simulink model "walkingRobot3DPath"  (R2022a)
settings: Solver=ode15s  StartTime=0.0  StopTime=70  RelTol=1e-2  EnableMultiTasking=on
PreLoadFcn:
  | robotParametersCtrl
values from neighbouring files (symbols this model uses):
  foot_x = 5    [robotParametersCtrl.m]
  foot_y = 4    [robotParametersCtrl.m]
  g = 9.80665    [robotParametersCtrl.m]
  h = 18    [robotParametersCtrl.m]
  Kwalk = 0.5    [robotParametersCtrl.m]
  stepHeight = 0.02    [robotParametersCtrl.m]
  torso_offset_z = -2    [robotParametersCtrl.m]
  TsCtrl = 0.05    [robotParametersCtrl.m]
  tWalk = 0.3    [robotParametersCtrl.m]
libraries: walkingRobotUtils x6, simulink x2, slpidlib x2
settings Model: Creator=scastro  LastModifiedBy=isamu
settings SolverCC: AlgebraicLoopSolver=TrustRegion
settings DataIOCC: ReturnWorkspaceOutputs=off  OutputTimes=0:0.01:10
settings OptimizationCC: LifeSpan=inf
settings DebuggingCC: UnconnectedInputMsg=warning  UnconnectedOutputMsg=warning  UnconnectedLineMsg=warning  AllowSymbolicDim=off  SFUnexpectedBacktrackingDiag=warning  SFNoUnconditionalDefaultTransitionDiag=warning  SFExecutionAtInitializationDiag=none  SFMachineParentedDataDiag=warning  UnitsInconsistencyMsg=none  ArithmeticOperatorsInVariantConditions=warning
settings SFSimCC: SimUseLocalCustomCode=off  CustomCodeUndefinedFunction=UseInterfaceOnly
settings RTWCC: RTWUseLocalCustomCode=off
settings CodeAppCC: StateflowObjectComments=on
settings GRTTargetCC: TargetLangStandard=C89/C90 (ANSI)
settings ConfigComp: CovMetricSettings=dw  CovSaveCumulativeToWorkspaceVar=on  CovSaveSingleToWorkspaceVar=on  CovExternalEMLEnable=off  CovSFcnEnable=off
settings SimscapeCC: SimscapeNormalizeSystem=off  SimscapeLogOpenViewer=on  SimscapeLogLimitData=off  SimscapeLogDataHistory=10000
settings ConfigurationSet: Description=SimMechanics 2G
settings DiagnosticsConfigSet: SimMechanicsRigidlyBoundBlock=none
settings ExplorerConfigSet: InternalSimMechanicsExplorerSettings="<ExplorerConfiguration><canonicalview>default</canonicalview><AnimationSetting><BasePlaybackSpeed>1.0</BasePlaybackSpeed><PlaybackSpeedFactor>1.0</PlaybackSpeedFactor></AnimationSetting><TilePanel><TileInfo><Tiles Columns=\"1\" Count=\"1\" Rows=\"1\"><Column Weight=\"1\"/><Row Weight=\"1\"/><Tile Height=\"1\" Width=\"1\" X=\"0\" Y=\"0\"/></Tiles></TileInfo><SceneInfo><SceneViewer><BGColor><R>0.60000002384185791</R><G>0.60000002384185791</G><B>0.60000002384185791</B></BGColor><Camera><DoPerspective>off</DoPerspective><Position><X>7.18002534815406079</X><Y>-8.21011991112170847</Y><Z>8.33180938462712462</Z></Position><Center><X>1.10741005252516134</X><Y>-0.176829942633513204</Y><Z>0.646464709811595872</Z></Center><Up><X>-0.335329266167064488</X><Y>0.506481739462631531</Y><Z>0.79437430147428989</Z></Up><ViewLimDist>1</ViewLimDist><YLim>0.739205014828661411</YLim><XLim>1.12849377732657596</XLim></Camera></SceneViewer></SceneInfo></TilePanel><MechEditorPanel><Cameras/><GfxPanelCameraMap/><VideoCreator><PlaybackSpeedRatio>1.0</PlaybackSpeedRatio><FrameRate>30</FrameRate><VideoFormat>Motion JPEG AVI</VideoFormat><FrameSize>auto</FrameSize></VideoCreator></MechEditorPanel></ExplorerConfiguration>"

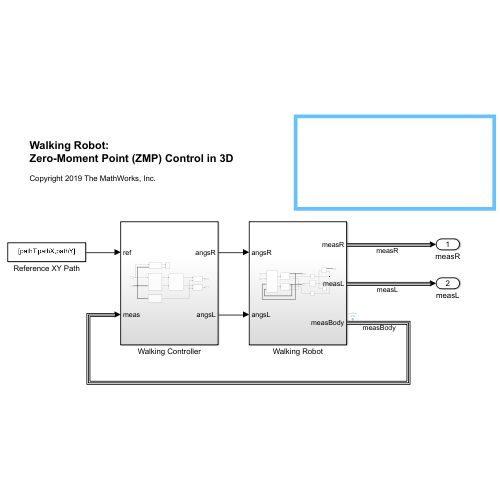
[thumbnail: Simulink's stored preview of the top-level diagram]
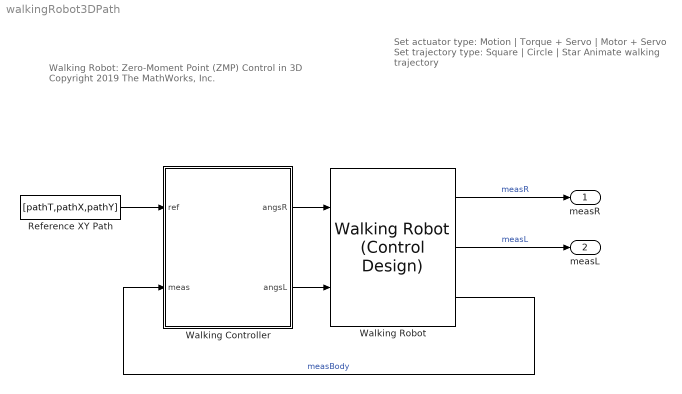
== system walkingRobot3DPath ==
  note: Set actuator type:
      | Motion | Torque + Servo | Motor + Servo
      |
      | Set trajectory type:
      | Square | Circle | Star
      |
      | Animate walking trajectory
  note: Walking Robot:
      | Zero-Moment Point (ZMP) Control in 3D
      |
      | Copyright 2019 The MathWorks, Inc.
  Reference XY Path : FromWorkspace  VariableName=[pathT,pathX,pathY]  SampleTime=TsCtrl  OutputAfterFinalValue=Holding final value
  Walking Controller : Subsystem
  Walking Robot : walkingRobotUtils/Walking Robot (Control Design)  SystemSampleTime=-1  VariantActivationTime=update diagram  Latency=0  AutoFrameSizeCalculation=off
  measR : Outport  VectorParamsAs1DForOutWhenUnconnected=off
  measL : Outport  Port=2  VectorParamsAs1DForOutWhenUnconnected=off
  wires:
  Walking Robot/1 -> measR/1  "measR"
  Walking Robot/2 -> measL/1  "measL"
  Walking Controller/1(angsR) -> Walking Robot/1
  Walking Controller/2(angsL) -> Walking Robot/2
  Walking Robot/3 -> Walking Controller/2(meas)  "measBody"
  Reference XY Path/1 -> Walking Controller/1(ref)

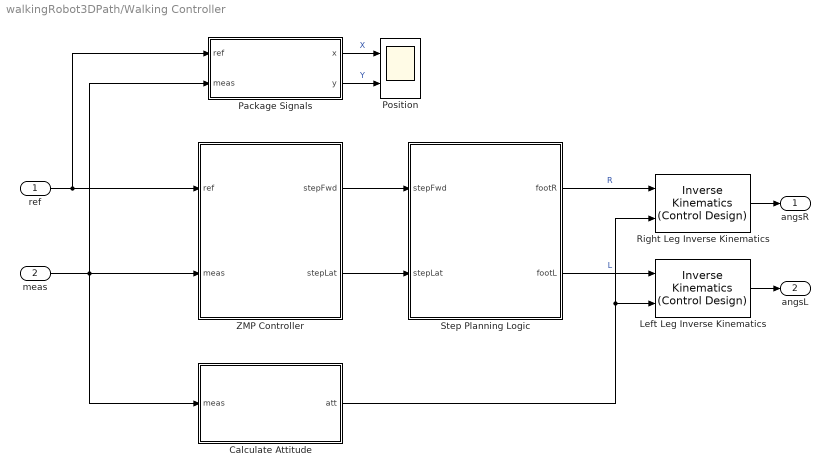
== system walkingRobot3DPath/Walking Controller ==
  ref : Inport
  meas : Inport  Port=2
  Calculate Attitude : Subsystem
  Left Leg Inverse Kinematics : walkingRobotUtils/Inverse Kinematics (Control Design)  SystemSampleTime=-1  VariantActivationTime=update diagram  Latency=0  AutoFrameSizeCalculation=off
  Package Signals : Subsystem
  Position : Scope  NumInputPorts=2
  Right Leg Inverse Kinematics : walkingRobotUtils/Inverse Kinematics (Control Design)  SystemSampleTime=-1  VariantActivationTime=update diagram  Latency=0  AutoFrameSizeCalculation=off
  Step Planning Logic : Stateflow chart  TreatAsAtomicUnit=on
  ZMP Controller : Subsystem
  angsR : Outport  VectorParamsAs1DForOutWhenUnconnected=off
  angsL : Outport  Port=2  VectorParamsAs1DForOutWhenUnconnected=off
  wires:
  ref/1 -> ZMP Controller/1(ref), Package Signals/1(ref)
  Right Leg Inverse Kinematics/1 -> angsR/1
  Left Leg Inverse Kinematics/1 -> angsL/1
  meas/1 -> Calculate Attitude/1(meas), Package Signals/2(meas), ZMP Controller/2("meas ")
  Package Signals/2(y) -> Position/2  "Y"
  Package Signals/1(x) -> Position/1  "X"
  Step Planning Logic/1(footR) -> Right Leg Inverse Kinematics/1  "R"
  Step Planning Logic/2(footL) -> Left Leg Inverse Kinematics/1  "L"
  ZMP Controller/1(stepFwd) -> Step Planning Logic/1(stepFwd)
  ZMP Controller/2(stepLat) -> Step Planning Logic/2(stepLat)
  Calculate Attitude/1(att) -> Left Leg Inverse Kinematics/2, Right Leg Inverse Kinematics/2

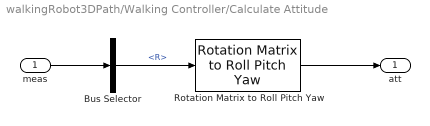
== system walkingRobot3DPath/Walking Controller/Calculate Attitude ==
  meas : Inport
  Bus Selector : BusSelector  OutputSignals=R
  Rotation Matrix to Roll Pitch Yaw : walkingRobotUtils/Rotation Matrix to  Roll Pitch Yaw  SystemSampleTime=-1  VariantActivationTime=update diagram  Latency=0  AutoFrameSizeCalculation=off
  att : Outport  VectorParamsAs1DForOutWhenUnconnected=off
  wires:
  Bus Selector/1 -> Rotation Matrix to Roll Pitch Yaw/1  "<R>"
  meas/1 -> Bus Selector/1
  Rotation Matrix to Roll Pitch Yaw/1 -> att/1

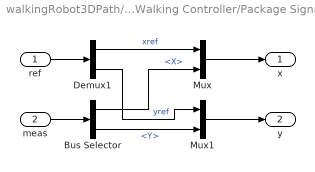
== system walkingRobot3DPath/Walking Controller/Package Signals ==
  ref : Inport
  meas : Inport  Port=2
  Bus Selector : BusSelector  OutputSignals=X,Y
  Demux1 : Demux  Outputs=2
  Mux : Mux  Inputs=2
  Mux1 : Mux  Inputs=2
  x : Outport  VectorParamsAs1DForOutWhenUnconnected=off
  y : Outport  Port=2  VectorParamsAs1DForOutWhenUnconnected=off
  wires:
  ref/1 -> Demux1/1
  Demux1/1 -> Mux/1  "xref"
  Bus Selector/2 -> Mux1/2  "<Y>"
  Mux/1 -> x/1
  meas/1 -> Bus Selector/1
  Bus Selector/1 -> Mux/2  "<X>"
  Mux1/1 -> y/1
  Demux1/2 -> Mux1/1  "yref"

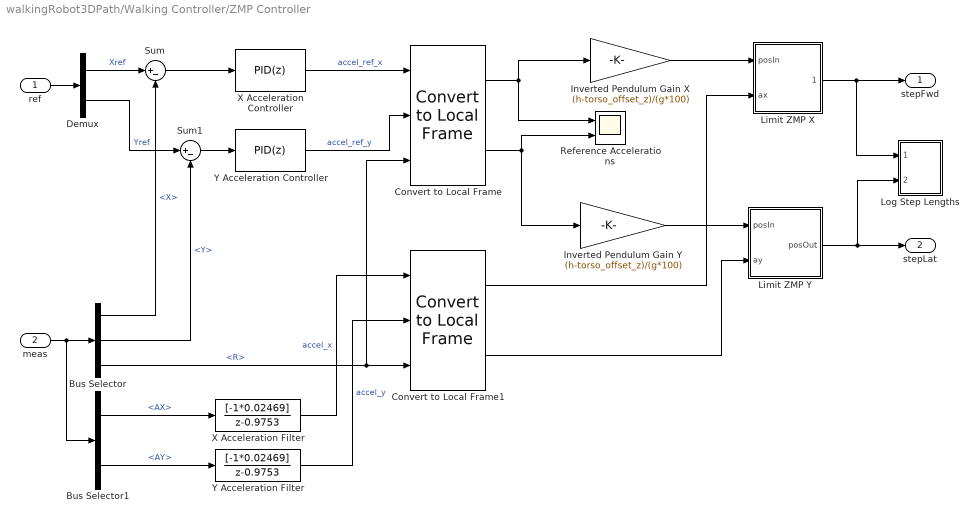
== system walkingRobot3DPath/Walking Controller/ZMP Controller ==
  ref : Inport
  "meas " : Inport  Port=2
  Bus Selector : BusSelector  OutputSignals=X,Y,R
  Bus Selector1 : BusSelector  OutputSignals=AX,AY
  Convert to Local Frame : walkingRobotUtils/Convert to Local Frame  SystemSampleTime=-1  VariantActivationTime=update diagram  Latency=0  AutoFrameSizeCalculation=off
  Convert to Local Frame1 : walkingRobotUtils/Convert to Local Frame  SystemSampleTime=-1  VariantActivationTime=update diagram  Latency=0  AutoFrameSizeCalculation=off
  Demux : Demux  Outputs=2
  Inverted Pendulum Gain X : Gain  Gain=(h-torso_offset_z)/(g*100)
  Inverted Pendulum Gain Y : Gain  Gain=(h-torso_offset_z)/(g*100)
  Limit ZMP X : Subsystem
  Limit ZMP Y : Subsystem
  Log Step Lengths : Subsystem
  Reference Accelerations : Scope  NumInputPorts=2
  Sum : Sum  Inputs=|+-
  Sum1 : Sum  Inputs=|+-
  X Acceleration Controller : slpidlib/PID Controller  Controller=PID  Form=Parallel  TimeDomain=Discrete-time  UseExternalTs=off  SampleTime=-1  IntegratorMethod=Forward Euler  FilterMethod=Forward Euler  ControllerParametersSource=internal  P=20  I=0  UseKiTs=off  D=2.5  N=0.5  UseFilter=on  TunerSelectOption=Transfer Function Based (PID Tuner App)  InitialConditionSource=internal  InitialConditionForIntegrator=0  InitialConditionForFilter=0  DifferentiatorICPrevScaledInput=0  ExternalReset=none  TrackingMode=off  Kt=1  LimitOutput=off  SatLimitsSource=internal  UpperSaturationLimit=inf  LowerSaturationLimit=-inf  LinearizeAsGain=off  AntiWindupMode=none  Kb=1  POutMin=[]  POutMax=[]  IOutMin=[]  IOutMax=[]  DOutMin=[]  DOutMax=[]  NOutMin=[]  NOutMax=[]  SumOutMin=[]  SumOutMax=[]  SaturationOutMin=[]  SaturationOutMax=[]  PParamMin=[]  PParamMax=[]  IParamMin=[]  IParamMax=[]  DParamMin=[]  DParamMax=[]  NParamMin=[]  NParamMax=[]  KbParamMin=[]  KbParamMax=[]  KtParamMin=[]  KtParamMax=[]  KbOutMin=[]  KbOutMax=[]  KtOutMin=[]  KtOutMax=[]  IntegratorOutMin=[]  IntegratorOutMax=[]  FilterOutMin=[]  FilterOutMax=[]  SumI1OutMin=[]  SumI1OutMax=[]  SumI2OutMin=[]  SumI2OutMax=[]  SumI3OutMin=[]  SumI3OutMax=[]  SumI4OutMin=[]  SumI4OutMax=[]  SumDOutMin=[]  SumDOutMax=[]  DifferentiatorOutMin=[]  DifferentiatorOutMax=[]  FilterDiffOutCoefMin=[]  FilterDiffOutCoefMax=[]  ReciprocalOutMin=[]  ReciprocalOutMax=[]  SumDenOutMin=[]  SumDenOutMax=[]  SumNumOutMin=[]  SumNumOutMax=[]  DivideOutMin=[]  DivideOutMax=[]  UdiffTsProdOutMin=[]  UdiffTsProdOutMax=[]  NTsProdOutMin=[]  NTsProdOutMax=[]  UintegralTsProdOutMin=[]  UintegralTsProdOutMax=[]  UngainTsProdOutMin=[]  UngainTsProdOutMax=[]  IntegratorContinuousStateAttributes=''  IntegratorStateMustResolveToSignalObject=off  IntegratorRTWStateStorageClass=Auto  FilterContinuousStateAttributes=''  FilterStateMustResolveToSignalObject=off  FilterRTWStateStorageClass=Auto  ParallelPVariant=InternalParameters  IdealPVariant=Disabled  IVariant=InternalParameters  DVariant=InternalParameters  IntegratorVariant=Discrete  SatVariant=Disabled  AWVariant=Passthrough  PCopyVariant=Disabled  TRVariant=Disabled  FdbkBlocksVariant=Forward  IdealPFdbkVariant=Disabled  SatFdbkVariant=Disabled  DerivativeFilterVariant=ForwardEulerFilter  NVariant=InternalParameters  NCopyVariant=Disabled  FilterICVariant=InternalICsFilter  IntegratorICVariant=InternalICs  ExternalResetVariant=Disabled  TRSumVariant=Passthrough  SumFdbkVariant=Disabled  SumVariant=Sum_PID  TsampFilterVariant=InternalTs  TsampNgainVariant=Passthrough  TsampIntegralVariant=Passthrough  ExternalSaturationOutDataTypeStr=Inherit: Same as second input  aMode=0
  X Acceleration Filter : DiscreteTransferFcn  Numerator=[-1*0.02469]  Denominator=[1 -0.9753]
  Y Acceleration Controller : slpidlib/PID Controller  Controller=PID  Form=Parallel  TimeDomain=Discrete-time  UseExternalTs=off  SampleTime=-1  IntegratorMethod=Forward Euler  FilterMethod=Forward Euler  ControllerParametersSource=internal  P=20  I=0  UseKiTs=off  D=2.5  N=0.5  UseFilter=on  TunerSelectOption=Transfer Function Based (PID Tuner App)  InitialConditionSource=internal  InitialConditionForIntegrator=0  InitialConditionForFilter=0  DifferentiatorICPrevScaledInput=0  ExternalReset=none  TrackingMode=off  Kt=1  LimitOutput=off  SatLimitsSource=internal  UpperSaturationLimit=inf  LowerSaturationLimit=-inf  LinearizeAsGain=off  AntiWindupMode=none  Kb=1  POutMin=[]  POutMax=[]  IOutMin=[]  IOutMax=[]  DOutMin=[]  DOutMax=[]  NOutMin=[]  NOutMax=[]  SumOutMin=[]  SumOutMax=[]  SaturationOutMin=[]  SaturationOutMax=[]  PParamMin=[]  PParamMax=[]  IParamMin=[]  IParamMax=[]  DParamMin=[]  DParamMax=[]  NParamMin=[]  NParamMax=[]  KbParamMin=[]  KbParamMax=[]  KtParamMin=[]  KtParamMax=[]  KbOutMin=[]  KbOutMax=[]  KtOutMin=[]  KtOutMax=[]  IntegratorOutMin=[]  IntegratorOutMax=[]  FilterOutMin=[]  FilterOutMax=[]  SumI1OutMin=[]  SumI1OutMax=[]  SumI2OutMin=[]  SumI2OutMax=[]  SumI3OutMin=[]  SumI3OutMax=[]  SumI4OutMin=[]  SumI4OutMax=[]  SumDOutMin=[]  SumDOutMax=[]  DifferentiatorOutMin=[]  DifferentiatorOutMax=[]  FilterDiffOutCoefMin=[]  FilterDiffOutCoefMax=[]  ReciprocalOutMin=[]  ReciprocalOutMax=[]  SumDenOutMin=[]  SumDenOutMax=[]  SumNumOutMin=[]  SumNumOutMax=[]  DivideOutMin=[]  DivideOutMax=[]  UdiffTsProdOutMin=[]  UdiffTsProdOutMax=[]  NTsProdOutMin=[]  NTsProdOutMax=[]  UintegralTsProdOutMin=[]  UintegralTsProdOutMax=[]  UngainTsProdOutMin=[]  UngainTsProdOutMax=[]  IntegratorContinuousStateAttributes=''  IntegratorStateMustResolveToSignalObject=off  IntegratorRTWStateStorageClass=Auto  FilterContinuousStateAttributes=''  FilterStateMustResolveToSignalObject=off  FilterRTWStateStorageClass=Auto  ParallelPVariant=InternalParameters  IdealPVariant=Disabled  IVariant=InternalParameters  DVariant=InternalParameters  IntegratorVariant=Discrete  SatVariant=Disabled  AWVariant=Passthrough  PCopyVariant=Disabled  TRVariant=Disabled  FdbkBlocksVariant=Forward  IdealPFdbkVariant=Disabled  SatFdbkVariant=Disabled  DerivativeFilterVariant=ForwardEulerFilter  NVariant=InternalParameters  NCopyVariant=Disabled  FilterICVariant=InternalICsFilter  IntegratorICVariant=InternalICs  ExternalResetVariant=Disabled  TRSumVariant=Passthrough  SumFdbkVariant=Disabled  SumVariant=Sum_PID  TsampFilterVariant=InternalTs  TsampNgainVariant=Passthrough  TsampIntegralVariant=Passthrough  ExternalSaturationOutDataTypeStr=Inherit: Same as second input  aMode=0
  Y Acceleration Filter : DiscreteTransferFcn  Numerator=[-1*0.02469]  Denominator=[1 -0.9753]
  stepFwd : Outport  VectorParamsAs1DForOutWhenUnconnected=off
  stepLat : Outport  Port=2  VectorParamsAs1DForOutWhenUnconnected=off
  wires:
  Sum/1 -> X Acceleration Controller/1
  X Acceleration Controller/1 -> Convert to Local Frame/1  "accel_ref_x"
  Sum1/1 -> Y Acceleration Controller/1
  ref/1 -> Demux/1
  Demux/1 -> Sum/1  "Xref"
  Bus Selector/1 -> Sum/2  "<X>"
  Bus Selector/2 -> Sum1/2  "<Y>"
  Demux/2 -> Sum1/1  "Yref"
  Bus Selector/3 -> Convert to Local Frame/3, Convert to Local Frame1/3  "<R>"
  Convert to Local Frame/1 -> Reference Accelerations/1, Inverted Pendulum Gain X/1
  Convert to Local Frame/2 -> Inverted Pendulum Gain Y/1, Reference Accelerations/2
  "meas "/1 -> Bus Selector1/1, Bus Selector/1
  Bus Selector1/1 -> X Acceleration Filter/1  "<AX>"
  Bus Selector1/2 -> Y Acceleration Filter/1  "<AY>"
  X Acceleration Filter/1 -> Convert to Local Frame1/1  "accel_x"
  Y Acceleration Filter/1 -> Convert to Local Frame1/2  "accel_y"
  Inverted Pendulum Gain X/1 -> Limit ZMP X/1(posIn)
  Convert to Local Frame1/1 -> Limit ZMP X/2(ax)
  Inverted Pendulum Gain Y/1 -> Limit ZMP Y/1(posIn)
  Convert to Local Frame1/2 -> Limit ZMP Y/2(ay)
  Y Acceleration Controller/1 -> Convert to Local Frame/2  "accel_ref_y"
  Limit ZMP X/1(posOut) -> Log Step Lengths/1(stepFwd), stepFwd/1
  Limit ZMP Y/1(posOut) -> Log Step Lengths/2(stepLat), stepLat/1

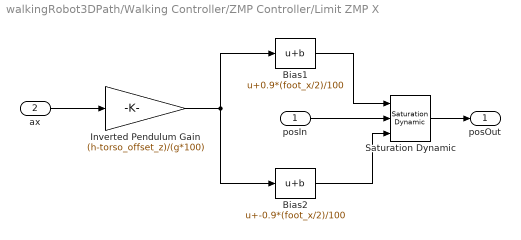
== system walkingRobot3DPath/Walking Controller/ZMP Controller/Limit ZMP X ==
  posIn : Inport
  ax : Inport  Port=2
  Bias1 : Bias  Bias=0.9*(foot_x/2)/100  SaturateOnIntegerOverflow=off
  Bias2 : Bias  Bias=-0.9*(foot_x/2)/100  SaturateOnIntegerOverflow=off
  Inverted Pendulum Gain : Gain  Gain=(h-torso_offset_z)/(g*100)
  Saturation Dynamic : simulink/Discontinuities/Saturation Dynamic  OutMin=[]  OutMax=[]  OutDataTypeStr=Inherit: Same as second input  OutDataType=fixdt(1, 16)  OutScaling=2^-10  DoSatur=off
  posOut : Outport  VectorParamsAs1DForOutWhenUnconnected=off
  wires:
  posIn/1 -> Saturation Dynamic/2
  Bias2/1 -> Saturation Dynamic/3
  Bias1/1 -> Saturation Dynamic/1
  ax/1 -> Inverted Pendulum Gain/1
  Saturation Dynamic/1 -> posOut/1
  Inverted Pendulum Gain/1 -> Bias1/1, Bias2/1

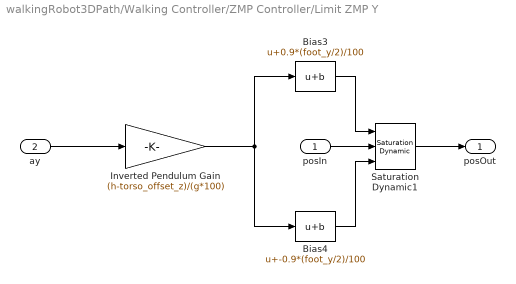
== system walkingRobot3DPath/Walking Controller/ZMP Controller/Limit ZMP Y ==
  posIn : Inport
  ay : Inport  Port=2
  Bias3 : Bias  Bias=0.9*(foot_y/2)/100  SaturateOnIntegerOverflow=off
  Bias4 : Bias  Bias=-0.9*(foot_y/2)/100  SaturateOnIntegerOverflow=off
  Inverted Pendulum Gain : Gain  Gain=(h-torso_offset_z)/(g*100)
  Saturation Dynamic1 : simulink/Discontinuities/Saturation Dynamic  OutMin=[]  OutMax=[]  OutDataTypeStr=Inherit: Same as second input  OutDataType=fixdt(1, 16)  OutScaling=2^-10  DoSatur=off
  posOut : Outport  VectorParamsAs1DForOutWhenUnconnected=off
  wires:
  Bias4/1 -> Saturation Dynamic1/3
  Bias3/1 -> Saturation Dynamic1/1
  Inverted Pendulum Gain/1 -> Bias4/1, Bias3/1
  ay/1 -> Inverted Pendulum Gain/1
  posIn/1 -> Saturation Dynamic1/2
  Saturation Dynamic1/1 -> posOut/1

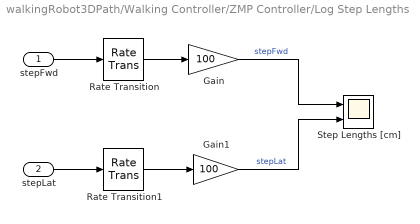
== system walkingRobot3DPath/Walking Controller/ZMP Controller/Log Step Lengths ==
  stepFwd : Inport
  stepLat : Inport  Port=2
  Gain : Gain  Gain=100
  Gain1 : Gain  Gain=100
  Rate Transition : RateTransition  OutPortSampleTime=tWalk
  Rate Transition1 : RateTransition  OutPortSampleTime=tWalk
  Step Lengths [cm] : Scope  NumInputPorts=2
  wires:
  Rate Transition/1 -> Gain/1
  Gain/1 -> Step Lengths [cm]/1  "stepFwd"
  Gain1/1 -> Step Lengths [cm]/2  "stepLat"
  stepFwd/1 -> Rate Transition/1
  Rate Transition1/1 -> Gain1/1
  stepLat/1 -> Rate Transition1/1

== stateflow chart walkingRobot3DPath/Walking Controller/Step Planning Logic ==
  settings: updateMethod=DISCRETE  sampleTime=TsCtrl
  state control [function]
    (default) -> (junction 43) : {
        | xR = xR + Kwalk*(xrefR-xR);
        | yR = yR + Kwalk*(yrefR-yR);
        | zR = zR + Kwalk*(zrefR-zR);
        | xL = xL + Kwalk*(xrefL-xL);
        | yL = yL + Kwalk*(yrefL-yL);
        | zL = zL + Kwalk*(zrefL-zL);
        | footR = [xR;yR;zR];
        | footL = [xL;yL;zL];
        | }
  state RightStep
    % Right foot is active
    % Left foot drags
    en, du:
    control;
    state RightFoot [parallel]
      en,du:
      zrefL = low;
      xrefR = stepFwd;
      yrefR = min(0,stepLat);
      zrefR = high;
      on after(0.5*tWalk,sec):
      zrefR = low;
      settings: executionOrder=1
    state LeftFoot [parallel]
      en,du:
      xrefL = -xrefR;
      yrefL = -min(stepLat,0);
      settings: executionOrder=2
  state LeftStep
    % Left foot is active
    % Right foot drags
    en, du:
    control;
    state RightFoot [parallel]
      en,du:
      xrefR = -xrefL;
      yrefR = -max(0,stepLat);
      settings: executionOrder=2
    state LeftFoot [parallel]
      en,du:
      zrefR = low;
      xrefL = stepFwd;
      yrefL = max(0,stepLat);
      zrefL = high;
      on after(0.5*tWalk,sec):
      zrefL = low;
      settings: executionOrder=1
  (default) -> RightStep : % Initialize values
      | {
      | low = -h/100;
      | high = low + stepHeight;
      | xL = 0; yL = 0; zL = low;
      | xR = 0; yR = 0; zR = low;
      | xrefL = 0; yrefL = 0; zrefL = low;
      | xrefR = 0; yrefR = 0; zrefR = low;
      | }
  RightStep -> LeftStep : [after(tWalk,sec)]
  LeftStep -> RightStep : [after(tWalk,sec)]
  data: footR output; footL output; stepFwd input; stepLat input; xR local; yR local; zR local; high local; xL local; yL local; zL local; low local; stepHeight parameter; h parameter; Kwalk parameter; yrefL local; zrefL local; xrefL local; yrefR local; zrefR local; xrefR local; tWalk parameter
